simulink library "DoorHndReq"  (R2022a)
settings: Solver=VariableStepAuto  StartTime=0.0  StopTime=10.0  RelTol=1e-3
settings Model: Creator=DELL  LastModifiedBy=DELL

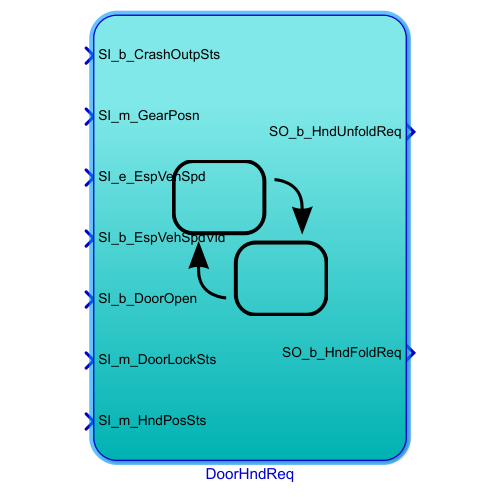
[thumbnail: Simulink's stored preview of the top-level diagram]
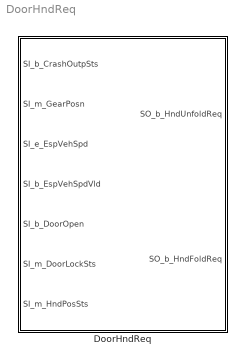
== system DoorHndReq ==
  DoorHndReq : Stateflow chart  TreatAsAtomicUnit=on

== stateflow chart DoorHndReq/DoorHndReq ==
  state PowerOnDelay
  state Func
    state Fold [parallel]
      settings: executionOrder=1
      state Idle
        (default) -> (junction 706) : {SO_b_HndFoldReq = 0;}
        Func.Fold.Idle -> (junction 706) [order 1]
        (junction 706) -> (junction 710) [order 1] : [SI_m_DoorLockSts != Door_Lock && ...
            | SI_e_EspVehSpd < 15]
        (junction 706) -> (junction 702) [order 2]
        (junction 710) -> (junction 703) : {SL_b_FoldReqTrig = 0;}
        (junction 703) -> (junction 702)
        (junction 702) -> (junction 707)
      state FoldReq
        en:
        SO_b_HndFoldReq = 1;
        SL_b_FoldReqTrig = 1;
      (default) -> Func.Fold.Idle
      Func.Fold.Idle -> FoldReq [order 1] : [(SI_m_DoorLockSts == Door_Lock || ...
          | SI_e_EspVehSpd >= 15) &&...
          | SL_b_FoldReqTrig == 0 && ...
          | SI_b_CrashOutpSts == 0 && ...
          | SI_m_HndPosSts != Hnd_Fold]
      FoldReq -> Func.Fold.Idle : [after(5, tick)]
    state Unfold [parallel]
      settings: executionOrder=2
      state Idle
        (default) -> (junction 687) : {SO_b_HndUnfoldReq = 0;}
        Func.Unfold.Idle -> (junction 687) [order 1]
        (junction 687) -> (junction 688) [order 1] : [SI_b_DoorOpen == 0 && ...
            | SI_m_DoorLockSts != Door_Unlock]
        (junction 687) -> (junction 689) [order 2]
        (junction 688) -> (junction 690) : {SL_b_UnfoldReqTrig = 0;}
        (junction 690) -> (junction 689)
        (junction 689) -> (junction 691)
      state NormalUnfoldReq
        en:
        SO_b_HndUnfoldReq = 1;
        SL_b_UnfoldReqTrig = 1;
      state CrashUnfoldReq
        en:
        SO_b_HndUnfoldReq = 1;
      (default) -> Func.Unfold.Idle
      Func.Unfold.Idle -> NormalUnfoldReq [order 1] : [SI_e_EspVehSpd < 15 && ...
          | (SI_b_DoorOpen == 1 || SI_m_DoorLockSts == Door_Unlock) && ...
          | SL_b_UnfoldReqTrig == 0 && ...
          | SI_m_HndPosSts != Hnd_Unfold]
      NormalUnfoldReq -> Func.Unfold.Idle : [after(5, tick)]
      Func.Unfold.Idle -> CrashUnfoldReq [order 2] : [hasChangedTo(SI_b_CrashOutpSts, 1) && ...
          | SI_m_HndPosSts != Hnd_Unfold]
      CrashUnfoldReq -> Func.Unfold.Idle : after(5, tick)
  state AntiPlay [commented out]
    state Count [commented out]
      (default) -> (junction 654) [commented out]
      Count -> (junction 654) [commented out]
      (junction 654) -> (junction 655) [commented out] : [hasChangedTo(SI_m_HndPosSts, Hnd_Fold) || ...
          | hasChangedTo(SI_m_HndPosSts, Hnd_Unfold)]
      (junction 654) -> (junction 656) [commented out]
      (junction 655) -> (junction 662) [commented out] : {SL_e_antiPlayCount++;}
      (junction 662) -> (junction 656) [commented out]
      (junction 656) -> (junction 658) [commented out]
    state TrigAndClean [commented out]
      en:
      SL_b_antiPlayFlg = 1;
      SL_e_antiPlayCount = 0;
    state Clean [commented out]
      en:
      SL_e_antiPlayCount = 0;
    (default) -> Count [commented out]
    Count -> TrigAndClean [commented out] : [before(3000, tick) &&...
        | SL_e_antiPlayCount >= 10]
    TrigAndClean -> Count [commented out] : [after(18000, tick)]
        | {SL_b_antiPlayFlg = 0;}
    Count -> Clean [commented out] : [after(3000, tick)]
    Clean -> Count [commented out]
  (default) -> PowerOnDelay
  PowerOnDelay -> Func : [after(100, tick)]
      | /* 上电延迟1s，防止底层信号量未及时传递导致请求误触发 */
  data: SI_b_CrashOutpSts input boolean; SI_m_GearPosn input Enum: Gear_Posn_E; SI_e_EspVehSpd input uint8; SI_b_EspVehSpdVld input boolean; SI_b_DoorOpen input boolean =0; SI_m_DoorLockSts input Enum: Door_Sts_E; SO_b_HndUnfoldReq output boolean; SL_e_antiPlayCount local uint8 =0; SI_m_HndPosSts input Enum: HndPos_Sts_E; SO_b_HndFoldReq output boolean; SL_b_antiPlayFlg local boolean =0; SL_b_UnfoldReqTrig local boolean =0; SL_b_FoldReqTrig local boolean =0
